simulink model "DIMR_ordinary"  (R2024b)
settings: Solver=daessc  StartTime=0.0  StopTime=60  RelTol=1e-3
values from neighbouring files (symbols this model uses):
  d_m0 = d_mn    (= 0)    [DIMR_main.m]
  d_m_cmd = 0.12787808985686    (= 0.127878089857)    [DIMR_main.m]
  dis_cmd = 0    [DIMR_main.m]
  jrk_cmd = 0.15    [DIMR_main.m]
  phi_cmd = 0*pi/180    (= 0)    [DIMR_main.m]
  ta = (vel_cmd-jrk_cmd*tt^2)/acc_cmd    (= 3.66666666667)    [DIMR_main.m]
  taz = z_vel_cmd/z_acc_cmd    (= 1.6)    [DIMR_main.m]
  tc = (x_cmd-2*(1/2*acc_cmd*ta^2+1/2*jrk_cmd*tt^2*ta+tt*vel_cmd))/vel_cmd    (= 10.6666666667)    [DIMR_main.m]
  tcz = (z_cmd-z_acc_cmd*taz^2)/z_vel_cmd    [DIMR_main.m]
  tcz2 = (z_cmd2-z_acc_cmd*taz^2)/z_vel_cmd    (= 0.9)    [DIMR_main.m]
  theta_f0 = -theta_p0    (= -0.024)    [DIMR_main.m]
  theta_f_cmd = 0.037940459    [DIMR_main.m]
  theta_p0 = theta_pn    (= 0.024)    [DIMR_main.m]
  theta_p_cmd = -0.037940459    [DIMR_main.m]
  ts = 15    [DIMR_main.m]
  ts2 = te+5    (= 39.3333333333)    [DIMR_main.m]
  tsz = 10    [DIMR_main.m]
  tsz2 = ts2    (= 39.3333333333)    [DIMR_main.m]
  tt = acc_cmd/jrk_cmd    (= 0.333333333333)    [DIMR_main.m]
  x_cmd = 3    [DIMR_main.m]
  z_0 = R_wo+L_bmy+L_my/2    [DIMR_main.m]
  z_acc_cmd = 0.05    [DIMR_main.m]
  z_cmd = 0.9-z_0    [DIMR_main.m]
  z_cmd2 = 0.9-0.7    (= 0.2)    [DIMR_main.m]
undefined symbols (not defined in the file or in its folder): Ac, Dc, DiscIntNeverNeededParam, dspblkCoreblockFVToolHelper, g, g_ext, g_fork, g_lift, g_reac, g_spado, g_yaw, gcbh, K_fd, K_fp, K_md, K_mp, K_pd, K_pp, K_wd, K_wi, K_wp, K_yd, K_yp, Kc, L_bg, L_bmx, L_bmy, L_bmz, L_bsx, L_bsy, L_bsz, L_by, L_ex, L_ey, L_ez, L_fg, L_fh, L_fx, L_fy, L_fz, L_lx, L_ly, L_lz, L_mg, L_mx, L_my, L_mz, L_wt, M_b, M_f, M_m, M_n11, M_n21, M_n22, M_n33, M_n44, Mc, N_f, N_w, omega_c ... (+10)
libraries: simulink x56, sm_lib x54, nesl_utility x12, slctrl_autotuning x1, slpidlib x1
(part 6 of 6)

== matlab function DIMR_ordinary/simp_model ==
  data: inv_cog_theta1 output; lt input; mass_l input; tau input; tau_w input; inv_cog_delta2 output; inv_cog_dtheta1 output; inv_cog_ddelta2 output
function [inv_cog_theta1,inv_cog_delta2,inv_cog_dtheta1,inv_cog_ddelta2] = simp_model(lt,mass_l,tau,tau_w)
%#codegen

%    This function was generated by the Symbolic Math Toolbox version 24.2.
%    16-Apr-2025 15:03:53

% lt = complex(lt);  % if required to enforce complex operations
% mass_l = complex(mass_l);  % if required to enforce complex operations
% tau = complex(tau);  % if required to enforce complex operations
% tau_w = complex(tau_w);  % if required to enforce complex operations
t0 = roots([tau.*-4.786091217110344e+34-tau.*tan(atan(((lt.*3.671450002392298e+16-sqrt(lt.^2.*1.34795451200664e+33-tau_w.^2.*3.022314549036573e+27+lt.^2.*tau_w.^2.*4.75626088156714e+29)).*4.447070890666667e+5)./(tau_w.*2.444803076916086e+19-lt.*tau_w.*3.066951346239308e+20)).*2.0).^2.*4.786091217110344e+34-tan(atan(((lt.*3.671450002392298e+16-sqrt(lt.^2.*1.34795451200664e+33-tau_w.^2.*3.022314549036573e+27+lt.^2.*tau_w.^2.*4.75626088156714e+29)).*4.447070890666667e+5)./(tau_w.*2.444803076916086e+19-lt.*tau_w.*3.066951346239308e+20)).*2.0).^2.*1.807017575219593e+35+lt.^2.*tan(atan(((lt.*3.671450002392298e+16-sqrt(lt.^2.*1.34795451200664e+33-tau_w.^2.*3.022314549036573e+27+lt.^2.*tau_w.^2.*4.75626088156714e+29)).*4.447070890666667e+5)./(tau_w.*2.444803076916086e+19-lt.*tau_w.*3.066951346239308e+20)).*2.0).^2.*1.413432750381875e+39-tau.^2.*tan(atan(((lt.*3.671450002392298e+16-sqrt(lt.^2.*1.34795451200664e+33-tau_w.^2.*3.022314549036573e+27+lt.^2.*tau_w.^2.*4.75626088156714e+29)).*4.447070890666667e+5)./(tau_w.*2.444803076916086e+19-lt.*tau_w.*3.066951346239308e+20)).*2.0).^2.*3.169126500570574e+33-tau.^2.*3.169126500570574e+33+lt.^2.*mass_l.*tan(atan(((lt.*3.671450002392298e+16-sqrt(lt.^2.*1.34795451200664e+33-tau_w.^2.*3.022314549036573e+27+lt.^2.*tau_w.^2.*4.75626088156714e+29)).*4.447070890666667e+5)./(tau_w.*2.444803076916086e+19-lt.*tau_w.*3.066951346239308e+20)).*2.0).^2.*4.151050661914464e+37+lt.^2.*mass_l.^2.*tan(atan(((lt.*3.671450002392298e+16-sqrt(lt.^2.*1.34795451200664e+33-tau_w.^2.*3.022314549036573e+27+lt.^2.*tau_w.^2.*4.75626088156714e+29)).*4.447070890666667e+5)./(tau_w.*2.444803076916086e+19-lt.*tau_w.*3.066951346239308e+20)).*2.0).^2.*3.047761132095789e+35-1.807017575219593e+35,lt.^2.*tan(atan(((lt.*3.671450002392298e+16-sqrt(lt.^2.*1.34795451200664e+33-tau_w.^2.*3.022314549036573e+27+lt.^2.*tau_w.^2.*4.75626088156714e+29)).*4.447070890666667e+5)./(tau_w.*2.444803076916086e+19-lt.*tau_w.*3.066951346239308e+20)).*2.0).*5.653731001527501e+39+lt.^2.*mass_l.^2.*tan(atan(((lt.*3.671450002392298e+16-sqrt(lt.^2.*1.34795451200664e+33-tau_w.^2.*3.022314549036573e+27+lt.^2.*tau_w.^2.*4.75626088156714e+29)).*4.447070890666667e+5)./(tau_w.*2.444803076916086e+19-lt.*tau_w.*3.066951346239308e+20)).*2.0).*1.219104452838316e+36+lt.^2.*mass_l.*tan(atan(((lt.*3.671450002392298e+16-sqrt(lt.^2.*1.34795451200664e+33-tau_w.^2.*3.022314549036573e+27+lt.^2.*tau_w.^2.*4.75626088156714e+29)).*4.447070890666667e+5)./(tau_w.*2.444803076916086e+19-lt.*tau_w.*3.066951346239308e+20)).*2.0).*1.660420264765786e+38,tau.*9.572182434220687e+34+tau.*tan(atan(((lt.*3.671450002392298e+16-sqrt(lt.^2.*1.34795451200664e+33-tau_w.^2.*3.022314549036573e+27+lt.^2.*tau_w.^2.*4.75626088156714e+29)).*4.447070890666667e+5)./(tau_w.*2.444803076916086e+19-lt.*tau_w.*3.066951346239308e+20)).*2.0).^2.*9.572182434220687e+34+tan(atan(((lt.*3.671450002392298e+16-sqrt(lt.^2.*1.34795451200664e+33-tau_w.^2.*3.022314549036573e+27+lt.^2.*tau_w.^2.*4.75626088156714e+29)).*4.447070890666667e+5)./(tau_w.*2.444803076916086e+19-lt.*tau_w.*3.066951346239308e+20)).*2.0).^2.*3.614035150439186e+35+lt.^2.*mass_l.*1.660420264765786e+38-lt.^2.*tan(atan(((lt.*3.671450002392298e+16-sqrt(lt.^2.*1.34795451200664e+33-tau_w.^2.*3.022314549036573e+27+lt.^2.*tau_w.^2.*4.75626088156714e+29)).*4.447070890666667e+5)./(tau_w.*2.444803076916086e+19-lt.*tau_w.*3.066951346239308e+20)).*2.0).^2.*2.82686550076375e+39+tau.^2.*tan(atan(((lt.*3.671450002392298e+16-sqrt(lt.^2.*1.34795451200664e+33-tau_w.^2.*3.022314549036573e+27+lt.^2.*tau_w.^2.*4.75626088156714e+29)).*4.447070890666667e+5)./(tau_w.*2.444803076916086e+19-lt.*tau_w.*3.066951346239308e+20)).*2.0).^2.*6.338253001141147e+33+lt.^2.*5.653731001527501e+39+tau.^2.*6.338253001141147e+33+lt.^2.*mass_l.^2.*1.219104452838316e+36-lt.^2.*mass_l.*tan(atan(((lt.*3.671450002392298e+16-sqrt(lt.^2.*1.34795451200664e+33-tau_w.^2.*3.022314549036573e+27+lt.^2.*tau_w.^2.*4.75626088156714e+29)).*4.447070890666667e+5)./(tau_w.*2.444803076916086e+19-lt.*tau_w.*3.066951346239308e+20)).*2.0).^2.*8.302101323828929e+37-lt.^2.*mass_l.^2.*tan(atan(((lt.*3.671450002392298e+16-sqrt(lt.^2.*1.34795451200664e+33-tau_w.^2.*3.022314549036573e+27+lt.^2.*tau_w.^2.*4.75626088156714e+29)).*4.447070890666667e+5)./(tau_w.*2.444803076916086e+19-lt.*tau_w.*3.066951346239308e+20)).*2.0).^2.*6.095522264191578e+35+3.614035150439186e+35,lt.^2.*tan(atan(((lt.*3.671450002392298e+16-sqrt(lt.^2.*1.34795451200664e+33-tau_w.^2.*3.022314549036573e+27+lt.^2.*tau_w.^2.*4.75626088156714e+29)).*4.447070890666667e+5)./(tau_w.*2.444803076916086e+19-lt.*tau_w.*3.066951346239308e+20)).*2.0).*-5.653731001527501e+39-lt.^2.*mass_l.^2.*tan(atan(((lt.*3.671450002392298e+16-sqrt(lt.^2.*1.34795451200664e+33-tau_w.^2.*3.022314549036573e+27+lt.^2.*tau_w.^2.*4.75626088156714e+29)).*4.447070890666667e+5)./(tau_w.*2.444803076916086e+19-lt.*tau_w.*3.066951346239308e+20)).*2.0).*1.219104452838316e+36-lt.^2.*mass_l.*tan(atan(((lt.*3.671450002392298e+16-sqrt(lt.^2.*1.34795451200664e+33-tau_w.^2.*3.022314549036573e+27+lt.^2.*tau_w.^2.*4.75626088156714e+29)).*4.447070890666667e+5)./(tau_w.*2.444803076916086e+19-lt.*tau_w.*3.066951346239308e+20)).*2.0).*1.660420264765786e+38,tau.*-4.786091217110344e+34-tau.*tan(atan(((lt.*3.671450002392298e+16-sqrt(lt.^2.*1.34795451200664e+33-tau_w.^2.*3.022314549036573e+27+lt.^2.*tau_w.^2.*4.75626088156714e+29)).*4.447070890666667e+5)./(tau_w.*2.444803076916086e+19-lt.*tau_w.*3.066951346239308e+20)).*2.0).^2.*4.786091217110344e+34-tan(atan(((lt.*3.671450002392298e+16-sqrt(lt.^2.*1.34795451200664e+33-tau_w.^2.*3.022314549036573e+27+lt.^2.*tau_w.^2.*4.75626088156714e+29)).*4.447070890666667e+5)./(tau_w.*2.444803076916086e+19-lt.*tau_w.*3.066951346239308e+20)).*2.0).^2.*1.807017575219593e+35+lt.^2.*tan(atan(((lt.*3.671450002392298e+16-sqrt(lt.^2.*1.34795451200664e+33-tau_w.^2.*3.022314549036573e+27+lt.^2.*tau_w.^2.*4.75626088156714e+29)).*4.447070890666667e+5)./(tau_w.*2.444803076916086e+19-lt.*tau_w.*3.066951346239308e+20)).*2.0).^2.*1.413432750381875e+39-tau.^2.*tan(atan(((lt.*3.671450002392298e+16-sqrt(lt.^2.*1.34795451200664e+33-tau_w.^2.*3.022314549036573e+27+lt.^2.*tau_w.^2.*4.75626088156714e+29)).*4.447070890666667e+5)./(tau_w.*2.444803076916086e+19-lt.*tau_w.*3.066951346239308e+20)).*2.0).^2.*3.169126500570574e+33-tau.^2.*3.169126500570574e+33+lt.^2.*mass_l.*tan(atan(((lt.*3.671450002392298e+16-sqrt(lt.^2.*1.34795451200664e+33-tau_w.^2.*3.022314549036573e+27+lt.^2.*tau_w.^2.*4.75626088156714e+29)).*4.447070890666667e+5)./(tau_w.*2.444803076916086e+19-lt.*tau_w.*3.066951346239308e+20)).*2.0).^2.*4.151050661914464e+37+lt.^2.*mass_l.^2.*tan(atan(((lt.*3.671450002392298e+16-sqrt(lt.^2.*1.34795451200664e+33-tau_w.^2.*3.022314549036573e+27+lt.^2.*tau_w.^2.*4.75626088156714e+29)).*4.447070890666667e+5)./(tau_w.*2.444803076916086e+19-lt.*tau_w.*3.066951346239308e+20)).*2.0).^2.*3.047761132095789e+35-1.807017575219593e+35]);
if tau_w >= 0
    t2 = real(t0(4));
else
    t2 = real(t0(3));
end
inv_cog_theta1 = atan(t2).*2.0;
if nargout > 1
    t3 = lt.^2;
    t4 = mass_l.^2;
    t5 = t2.^2;
    t6 = t2.^3;
    t7 = tau.^2;
    t8 = tau_w.^2;
    t9 = tau_w.*4.0e+2;
    t10 = lt.*3.671450002392298e+16;
    t14 = lt.*tau_w.*5.017911463213649e+3;
    t11 = t8.*3.022314549036573e+27;
    t13 = t3.*1.34795451200664e+33;
    t15 = -t14;
    t18 = t3.*t8.*4.75626088156714e+29;
    t12 = -t11;
    t16 = t9+t15;
    t17 = 1.0./t16;
    t19 = t12+t13+t18;
    t20 = sqrt(t19);
    t21 = -t20;
    t22 = t10+t21;
    t23 = (t17.*t22)./1.37438953472e+11;
    t24 = atan(t23);
    t25 = t24.*2.0;
    t26 = tan(t25);
    t27 = t26.^2;
    t28 = t26.^3;
    et1 = mass_l.*7.462747908049749e+36+t2.*2.168421090263512e+37-t6.*7.228070300878373e+36+t26.*7.228070300878373e+36;
    et2 = t27.*3.210929424600914e+38+t28.*7.228070300878373e+36+tau.*4.252255575316159e+37+mass_l.*t27.*7.462747908049749e+36;
    et3 = mass_l.*tau.*9.882967578188891e+35+t2.*t3.*2.261492400611e+41+t2.*t7.*3.802951800684688e+35-t6.*t7.*1.267650600228229e+35;
    et4 = t2.*t27.*2.168421090263512e+37-t3.*t26.*1.1307462003055e+41-t3.*t28.*5.653731001527501e+40-t5.*t26.*7.228070300878373e+36;
    et5 = t5.*t28.*-7.228070300878373e+36-t6.*t27.*7.228070300878373e+36+t7.*t26.*1.267650600228229e+35+t7.*t28.*1.267650600228229e+35;
    et6 = tau.*t2.*5.743309460532412e+36-t6.*tau.*1.914436486844137e+36+t26.*tau.*1.914436486844137e+36+t27.*tau.*4.252255575316159e+37;
    et7 = t28.*tau.*1.914436486844137e+36+mass_l.*t2.*t3.*6.641681059063143e+39-mass_l.*t3.*t26.*3.320840529531572e+39-mass_l.*t3.*t28.*1.660420264765786e+39;
    et8 = mass_l.*t27.*tau.*9.882967578188891e+35+t2.*t3.*t4.*4.876417811353262e+37+t2.*t3.*t27.*5.653731001527501e+40-t3.*t4.*t26.*2.438208905676631e+37;
    et9 = t3.*t5.*t26.*2.261492400611e+41-t3.*t4.*t28.*1.219104452838316e+37+t2.*t7.*t27.*3.802951800684688e+35+t3.*t5.*t28.*5.653731001527501e+40;
    et10 = t3.*t6.*t27.*5.653731001527501e+40-t5.*t7.*t26.*1.267650600228229e+35-t5.*t7.*t28.*1.267650600228229e+35-t6.*t7.*t27.*1.267650600228229e+35;
    et11 = t2.*t27.*tau.*5.743309460532412e+36-t5.*t26.*tau.*1.914436486844137e+36-t5.*t28.*tau.*1.914436486844137e+36-t6.*t27.*tau.*1.914436486844137e+36;
    et12 = mass_l.*t2.*t3.*t27.*1.660420264765786e+39+mass_l.*t3.*t5.*t26.*6.641681059063143e+39+mass_l.*t3.*t5.*t28.*1.660420264765786e+39+mass_l.*t3.*t6.*t27.*1.660420264765786e+39;
    et13 = t2.*t3.*t4.*t27.*1.219104452838316e+37+t3.*t4.*t5.*t26.*4.876417811353262e+37+t3.*t4.*t5.*t28.*1.219104452838316e+37+t3.*t4.*t6.*t27.*1.219104452838316e+37;
    et14 = 3.210929424600914e+38;
    inv_cog_delta2 = ((et1+et2+et3+et4+et5+et6+et7+et8+et9+et10+et11+et12+et13+et14).*(-2.264224836463332e-20))./((mass_l+2.5e+1).*(tau.*5.62949953421312e+16+4.250902933753714e+17).*(t27+1.0));
end
if nargout > 2
    inv_cog_dtheta1 = 0.0;
end
if nargout > 3
    inv_cog_ddelta2 = 0.0;
end
end

== stateflow chart DIMR_ordinary/Chart ==
  state Change_Height_1
    entry:
    [theta1,delta2,dtheta1,ddelta2,lt] = IK(dz,tau,z)
    during:
    [theta1,delta2,dtheta1,ddelta2,lt] = IK(dz,tau,z)
  state Move
    entry:
    [theta1,delta2,dtheta1,ddelta2] = simp_model(lt,tau,tau_w)
    during:
    [theta1,delta2,dtheta1,ddelta2] = simp_model(lt,tau,tau_w)
  (default) -> Change_Height_1
  Change_Height_1 -> Move : [abs(z_curr - z_cmd)<=0.001]
  data: dz function_input; tau function_input; z function_input; ik_theta1 function_output; ik_delta2 function_output; ik_dtheta1 function_output; ik_ddelta2 function_output; ik_lt function_output; lt function_input; tau function_input; tau_w function_input; inv_cog_theta1 function_output; inv_cog_delta2 function_output; inv_cog_dtheta1 function_output; inv_cog_ddelta2 function_output; tau_w input; z input; dz input; z_curr input; ddelta2 output; delta2 output; dtheta1 output; theta1 output; lt local; z_cmd input double; tau input
  function [ik_theta1,ik_delta2,ik_dtheta1,ik_ddelta2,ik_lt] = IK(dz,tau,z):
    | function [ik_theta1,ik_delta2,ik_dtheta1,ik_ddelta2,ik_lt] = IK(dz,tau,z)
    | %#codegen
    | 
    | %    This function was generated by the Symbolic Math Toolbox version 24.2.
    | %    15-Apr-2025 18:25:07
    | 
    | % dz = complex(dz);  % if required to enforce complex operations
    | % tau = complex(tau);  % if required to enforce complex operations
    | % z = complex(z);  % if required to enforce complex operations
    | t0 = roots([1.0,(tau.*8.44424930131968e+16-z.*6.07271847679102e+19-tau.*z.*1.125899906842624e+18+2.195986091984785e+19)./(tau.*1.238489897526886e+17+9.351986454258171e+17),0.0,((tau.*-8.44424930131968e+16+z.*6.07271847679102e+19+tau.*z.*1.125899906842624e+18+1.285078320466132e+19).*(-1.0./4.4e+2))./(tau.*2.81474976710656e+14+2.125451466876857e+15),-1.0]);
    | t2 = real(t0(4));
    | t3 = atan2(t2,1);
    | t4 = t2.^2;
    | t5 = t2.^3;
    | t6 = tau.^2;
    | t7 = tau.^3;
    | t9 = tau.^5;
    | t11 = z.^2;
    | t12 = z.^3;
    | t14 = z.^5;
    | t19 = tau.*1.40737488355328e+14;
    | t20 = tau.*5.319877059831398e+17;
    | t21 = t2.*tau.*1.238489897526886e+17;
    | t22 = t2.*9.351986454258171e+17;
    | t23 = tau.*z.*1.125899906842624e+18;
    | t24 = z.*6.07271847679102e+19;
    | t35 = tau.*4.635073695354219e-1;
    | t57 = tau.*5.743900035854321e+113;
    | t66 = tau.*z.*7.990597029423474e+114;
    | t74 = z.*1.447317376015955e+116;
    | t8 = t6.^2;
    | t10 = t6.^3;
    | t13 = t11.^2;
    | t15 = t11.^3;
    | t16 = t3.*2.0;
    | ik_theta1 = t16;
    | if nargout > 1
    |     t25 = -t23;
    |     t26 = -t24;
    |     t27 = t4.*tau.*8.44424930131968e+16;
    |     t28 = t5.*tau.*1.238489897526886e+17;
    |     t29 = t5.*9.351986454258171e+17;
    |     t30 = t4.*2.195986091984785e+19;
    |     t33 = t4.*tau.*z.*-1.125899906842624e+18;
    |     t34 = t4.*z.*-6.07271847679102e+19;
    |     t36 = t19+7.590898095988775e+15;
    |     t38 = t35+7.0./2.0;
    |     t39 = t35+6.81e+2./1.0e+1;
    |     t42 = t9.*2.386050182016105e+106;
    |     t46 = t9.*z.*4.211088297564564e+107;
    |     t51 = t7.*2.507343178421252e+110;
    |     t52 = t9.*t11.*4.593987726794744e+108;
    |     t58 = t9.*t12.*2.604615627247899e+109;
    |     t60 = t6.*2.999842761429269e+112;
    |     t61 = t7.*z.*9.409126505705104e+111;
    |     t65 = t9.*t14.*2.966510080312107e+110;
    |     t72 = -t66;
    |     t73 = t6.*z.*3.660741181676567e+113;
    |     t75 = t7.*t11.*6.407841099867219e+112;
    |     t76 = t7.*t12.*3.958710038416369e+112;
    |     t81 = -t74;
    |     t86 = t11.*tau.*3.585353509436109e+115;
    |     t87 = t6.*t11.*2.09113906624741e+114;
    |     t88 = t6.*t12.*3.785302651403782e+114;
    |     t90 = t7.*t14.*2.876678343420641e+114;
    |     t92 = t11.*7.09032593341523e+116;
    |     t93 = t12.*tau.*2.133985804221304e+116;
    |     t95 = t12.*3.242008287042286e+117;
    |     t98 = t14.*2.256895254686051e+118;
    |     t101 = t14.*tau.*2.510610198759619e+117;
    |     t102 = t6.*t14.*1.163686329155874e+116;
    |     t17 = cos(t16);
    |     t18 = sin(t16);
    |     t37 = 1.0./t36;
    |     t40 = 1.0./t39.^2;
    |     t41 = t10.*3.212055390272792e+104;
    |     t43 = t10.*z.*2.675474179773727e+105;
    |     t44 = t8.*2.477746168797788e+107;
    |     t47 = t10.*t11.*2.526492816377412e+106;
    |     t48 = -t46;
    |     t49 = t10.*t12.*1.059207781794524e+107;
    |     t50 = t10.*t13.*4.676525342669896e+107;
    |     t54 = t10.*t14.*9.166661893505187e+107;
    |     t55 = t10.*t15.*2.037035976334486e+108;
    |     t56 = t8.*z.*9.736596647488009e+109;
    |     t63 = -t58;
    |     t64 = t9.*t13.*1.239018969121646e+110;
    |     t67 = -t61;
    |     t68 = t8.*t11.*7.882227863274746e+110;
    |     t69 = t8.*t12.*2.154890938178742e+111;
    |     t70 = -t65;
    |     t71 = t9.*t15.*6.592244622915794e+110;
    |     t78 = t8.*t13.*1.21830758387732e+112;
    |     t79 = t8.*t14.*4.00008483587525e+112;
    |     t80 = -t73;
    |     t82 = -t76;
    |     t83 = t7.*t13.*4.915417942081258e+113;
    |     t85 = t8.*t15.*8.88907741305611e+112;
    |     t89 = t6.*t13.*1.928403609769147e+114;
    |     t91 = t7.*t15.*6.392618540934758e+114;
    |     t94 = t13.*tau.*3.97502326562149e+116;
    |     t96 = -t90;
    |     t97 = t13.*7.985575221783389e+117;
    |     t99 = t15.*5.015322788191225e+118;
    |     t103 = t6.*t15.*2.585969620346386e+116;
    |     t105 = -t98;
    |     t106 = -t101;
    |     t107 = t15.*tau.*5.579133775021375e+117;
    |     t108 = -t102;
    |     t109 = t20+t21+t22+t25+t26+t27+t28+t29+t30+t33+t34+2.869359480283757e+19;
    |     t45 = -t43;
    |     t53 = -t49;
    |     t59 = -t54;
    |     t62 = -t56;
    |     t77 = -t69;
    |     t84 = -t79;
    |     t100 = -t94;
    |     t104 = -t97;
    |     t110 = (t37.*t109)./8.0e+3;
    |     ik_delta2 = -t110;
    | end
    | if nargout > 2
    |     t111 = t110-1.59e+2./4.0e+2;
    |     t112 = t41+t42+t44+t45+t47+t48+t50+t51+t52+t53+t55+t57+t59+t60+t62+t63+t64+t67+t68+t70+t71+t72+t75+t77+t78+t80+t81+t82+t83+t84+t85+t86+t87+t88+t89+t91+t92+t93+t95+t96+t99+t100+t103+t104+t105+t106+t107+t108-2.105477541297374e+115;
    |     t113 = 1.0./t112;
    |     et1 = t2.*-1.753894605876528e+96+t4.*1.009464978528226e+96;
    |     et2 = t5.*4.619988807297373e+94-t6.*2.554852704393891e+92;
    |     et3 = t7.*-7.8111064788263e+89-t8.*1.00794759003273e+89;
    |     et4 = t9.*1.814387972119789e+86+t11.*6.245124509053326e+96;
    |     et5 = t12.*-3.331857083120826e+97;
    |     et6 = t13.*3.815554989087441e+97-tau.*5.24829876676123e+94;
    |     et7 = z.*1.399328629129073e+96-t2.*t6.*1.075720720231548e+91;
    |     et8 = t2.*t7.*-1.388092428471541e+90+t2.*t8.*7.128076116355089e+88;
    |     et9 = t4.*t6.*1.722969069981006e+93+t2.*t9.*1.361707336651519e+86;
    |     et10 = t4.*t7.*-1.973567476521639e+90+t5.*t6.*9.078257330103773e+92;
    |     et11 = t4.*t8.*1.151036106739522e+89+t5.*t7.*6.111449310419045e+90;
    |     et12 = t2.*t11.*5.875732481208788e+97+t4.*t9.*1.343184695804828e+87;
    |     et13 = t5.*t8.*-2.551325158332646e+88-t2.*t12.*1.782863198738202e+97;
    |     et14 = t5.*t9.*5.322204718218049e+86-t2.*t13.*5.464130766461227e+98;
    |     et15 = t4.*t11.*4.415911382468272e+97;
    |     et16 = t2.*t14.*8.258777032656798e+98;
    |     et17 = t4.*t12.*-8.469349253727501e+97;
    |     et18 = t5.*t11.*9.380726613532944e+95;
    |     et19 = t4.*t13.*6.359258315145734e+97;
    |     et20 = t5.*t12.*-1.175190936638932e+96+t6.*t11.*5.907708747848193e+94;
    |     et21 = t6.*t12.*-3.196898258866477e+95+t7.*t11.*1.247609721739556e+93;
    |     et22 = t6.*t13.*4.534279766579717e+95-t7.*t12.*6.544610701214467e+93;
    |     et23 = t8.*t11.*1.242487226117768e+91+t7.*t13.*1.139418916775499e+94;
    |     et24 = t8.*t12.*-5.845583673798496e+91+t9.*t11.*4.904790067467224e+88;
    |     et25 = t8.*t13.*1.333203858988986e+92-t9.*t12.*1.791158880389735e+89;
    |     et26 = t9.*t13.*5.970529601299116e+89+tau.*t2.*1.323988270291723e+93;
    |     et27 = t4.*tau.*1.468522013529346e+95+t5.*tau.*1.261219729665987e+94;
    |     et28 = t11.*tau.*1.207196483550789e+96;
    |     et29 = t12.*tau.*-6.477833809662083e+96;
    |     et30 = t13.*tau.*7.882625873837409e+96;
    |     et31 = z.*t2.*-1.890970205684437e+96;
    |     et32 = t4.*z.*-1.069218722198518e+97;
    |     et33 = t5.*z.*-3.150739272925472e+95+t6.*z.*2.668557352126731e+93;
    |     et34 = t7.*z.*4.092978643690637e+91+t8.*z.*6.846342443053817e+89;
    |     et35 = t9.*z.*-5.342131360762384e+87+tau.*z.*2.034429880145039e+95;
    |     et36 = t2.*t6.*t11.*3.834597488658114e+94+t2.*t6.*t12.*1.79267290146031e+95;
    |     et37 = t2.*t7.*t11.*3.241447763154754e+92-t2.*t6.*t13.*1.552786419763549e+96;
    |     et38 = t2.*t7.*t12.*4.397794916127146e+93+t2.*t8.*t11.*6.696326945473049e+89;
    |     et39 = t4.*t6.*t11.*2.979273638991897e+95;
    |     et40 = t2.*t6.*t14.*2.838892916716577e+96;
    |     et41 = t2.*t7.*t13.*-2.577198424443163e+94+t2.*t8.*t12.*4.358240682659937e+91;
    |     et42 = t2.*t9.*t11.*-1.748415316198616e+88-t4.*t6.*t12.*7.776982869967544e+95;
    |     et43 = t4.*t7.*t11.*4.360273950273173e+93+t5.*t6.*t11.*2.746751487155486e+94;
    |     et44 = t2.*t7.*t14.*5.263391152880169e+94-t2.*t8.*t13.*2.109408183024797e+92;
    |     et45 = t2.*t9.*t12.*1.455542746740951e+89+t4.*t6.*t13.*7.557132944299528e+95;
    |     et46 = t4.*t7.*t12.*-1.507615643654141e+94+t4.*t8.*t11.*2.876061807193666e+91;
    |     et47 = t5.*t6.*t12.*-3.913495645809803e+94+t5.*t7.*t11.*8.312588465463616e+92;
    |     et48 = t2.*t8.*t14.*4.879241176214998e+92-t2.*t9.*t13.*6.784692728748996e+89;
    |     et49 = t4.*t7.*t13.*1.899031527959165e+94-t4.*t8.*t12.*1.220393558543954e+92;
    |     et50 = t4.*t9.*t11.*1.010114099713122e+89-t5.*t7.*t12.*1.474838834239447e+93;
    |     et51 = t5.*t8.*t11.*9.289616355673145e+90+t2.*t9.*t14.*1.809251394333066e+90;
    |     et52 = t4.*t8.*t13.*2.22200643164831e+92-t4.*t9.*t12.*2.985264800649558e+89;
    |     et53 = t5.*t8.*t12.*-2.32376788561945e+91+t5.*t9.*t11.*2.955412152643063e+88;
    |     et54 = t4.*t9.*t13.*9.950882668831861e+89-t5.*t9.*t12.*1.313516512285806e+89;
    |     et55 = t2.*t11.*tau.*2.467684994491885e+96;
    |     et56 = t2.*t12.*tau.*2.151307797149133e+96;
    |     et57 = t2.*t13.*tau.*-4.626464408073966e+97;
    |     et58 = t4.*t11.*tau.*7.861141246672502e+96;
    |     et59 = t2.*t14.*tau.*7.65600803597262e+97;
    |     et60 = t4.*t12.*tau.*-1.628045107945128e+97;
    |     et61 = t5.*t11.*tau.*2.881458695288517e+95;
    |     et62 = t4.*t13.*tau.*1.313770978972902e+97;
    |     et63 = t5.*t12.*tau.*-3.766278218797084e+95-t2.*t6.*z.*8.69453683410162e+92;
    |     et64 = t2.*t7.*z.*-8.14011166039339e+90-t2.*t8.*z.*7.354331859382801e+89;
    |     et65 = t4.*t6.*z.*-4.607531607862968e+94-t2.*t9.*z.*1.094057710499569e+87;
    |     et66 = t4.*t7.*z.*-4.316771097086506e+92-t5.*t6.*z.*7.922329257005371e+93;
    |     et67 = t4.*t8.*z.*-2.629642166088229e+90-t5.*t7.*z.*1.751142096260925e+92;
    |     et68 = t4.*t9.*z.*-1.179328859496608e+88-t5.*t8.*z.*1.536226654469186e+90;
    |     et69 = t5.*t9.*z.*-8.573979033945596e+87-tau.*z.*t2.*1.644111357410597e+95;
    |     et70 = t4.*tau.*z.*-1.740373755123545e+96;
    |     et71 = t5.*tau.*z.*-9.219656825165702e+94-3.817418975922806e+95;
    |     ik_dtheta1 = dz.*t36.*t113.*(et1+et2+et3+et4+et5+et6+et7+et8+et9+et10+et11+et12+et13+et14+et15+et16+et17+et18+et19+et20+et21+et22+et23+et24+et25+et26+et27+et28+et29+et30+et31+et32+et33+et34+et35+et36+et37+et38+et39+et40+et41+et42+et43+et44+et45+et46+et47+et48+et49+et50+et51+et52+et53+et54+et55+et56+et57+et58+et59+et60+et61+et62+et63+et64+et65+et66+et67+et68+et69+et70+et71).*8.0e+3;
    | end
    | if nargout > 3
    |     et72 = t2.*-3.7071702195569e+114;
    |     et73 = t4.*3.804188113277026e+115;
    |     et74 = t5.*1.625202646823668e+114;
    |     et75 = t6.*1.140152959101139e+112;
    |     et76 = t7.*3.851536071140141e+109;
    |     et77 = t8.*4.771323709725432e+107;
    |     et78 = t9.*2.37036597763644e+105;
    |     et79 = t10.*3.344342724717159e+103;
    |     et80 = t11.*6.661710042517029e+116;
    |     et81 = t12.*3.317645224682185e+117;
    |     et82 = t13.*-8.033152579881287e+117+t55+t59+t70+t71+t84+t85+t91+t96+t99+t103+t105+t106+t107+t108;
    |     et83 = tau.*3.305389407105682e+113;
    |     et84 = z.*-1.344576683503948e+116;
    |     et85 = t2.*t6.*-5.521484071666565e+111;
    |     et86 = t2.*t7.*-1.201004210046715e+109;
    |     et87 = t2.*t8.*-1.446897405085628e+108;
    |     et88 = t4.*t6.*-7.600317735708989e+111;
    |     et89 = t2.*t9.*-6.836757611015585e+105;
    |     et90 = t4.*t7.*9.237917051294251e+109;
    |     et91 = t5.*t6.*-8.407795288014511e+110;
    |     et92 = t2.*t10.*4.905035996251834e+103;
    |     et93 = t4.*t8.*6.21766718480593e+107;
    |     et94 = t5.*t7.*-1.679675237605966e+109;
    |     et95 = t2.*t11.*2.425689270038724e+115;
    |     et96 = t4.*t9.*-2.369824972154481e+105;
    |     et97 = t5.*t8.*1.018828318361818e+108;
    |     et98 = t2.*t12.*-6.307571438901966e+116;
    |     et99 = t4.*t10.*3.344342724717159e+103;
    |     et100 = t5.*t9.*7.067802508371117e+105;
    |     et101 = t2.*t13.*1.396484281539863e+117;
    |     et102 = t4.*t11.*-1.402659673535802e+117;
    |     et103 = t5.*t10.*4.905035996251834e+103;
    |     et104 = t2.*t14.*-7.723597093814486e+116;
    |     et105 = t4.*t12.*3.938271388021781e+117;
    |     et106 = t5.*t11.*-5.533248821789028e+115;
    |     et107 = t4.*t13.*1.098783857622504e+118;
    |     et108 = t5.*t12.*1.557427551233363e+115;
    |     et109 = t6.*t11.*7.991271506884402e+113;
    |     et110 = t4.*t14.*-5.131828736560907e+118;
    |     et111 = t5.*t13.*5.110047691224071e+116;
    |     et112 = t6.*t12.*6.388892406797049e+114;
    |     et113 = t7.*t11.*2.225465716458933e+112;
    |     et114 = t5.*t14.*-7.723597093814486e+116;
    |     et115 = t6.*t13.*6.133630224665161e+112;
    |     et116 = t7.*t12.*6.414800515945154e+112;
    |     et117 = t8.*t11.*2.190420013370623e+110;
    |     et118 = t7.*t13.*4.024585580613185e+113;
    |     et119 = t8.*t12.*-3.271771400537028e+110;
    |     et120 = t9.*t11.*9.648630921792687e+107;
    |     et121 = t8.*t13.*1.013528935640283e+112;
    |     et122 = t9.*t12.*-1.235951960272058e+109;
    |     et123 = t10.*t11.*1.239367190298751e+106;
    |     et124 = t9.*t13.*1.011419526100604e+110;
    |     et125 = t10.*t12.*-7.63430158030757e+106;
    |     et126 = t10.*t13.*3.690599930124005e+107+t4.*t55+t4.*t71+t4.*t85+t4.*t91+t4.*t99+t4.*t103+t4.*t107;
    |     et127 = tau.*t2.*-5.325511928164662e+113;
    |     et128 = t4.*tau.*-4.601389533003556e+111;
    |     et129 = t5.*tau.*2.102524928619955e+113;
    |     et130 = t11.*tau.*2.257239068666816e+115;
    |     et131 = t12.*tau.*2.379035049732175e+116;
    |     et132 = t13.*tau.*-4.136321230248881e+116;
    |     et133 = z.*t2.*3.113201852556033e+115;
    |     et134 = t4.*z.*-6.511422436340579e+115;
    |     et135 = t5.*z.*1.662776353932113e+114;
    |     et136 = t6.*z.*-9.989623857325219e+112;
    |     et137 = t7.*z.*-3.096673052545432e+111;
    |     et138 = t8.*z.*-3.937587938067827e+109;
    |     et139 = t9.*z.*-6.92947223565074e+106;
    |     et140 = t10.*z.*-1.077535567389974e+105;
    |     et141 = tau.*z.*-4.956122630630957e+114;
    |     et142 = t2.*t6.*t11.*5.463288101128978e+113;
    |     et143 = t2.*t6.*t12.*-6.870842133918736e+114;
    |     et144 = t2.*t7.*t11.*1.493465513298907e+112;
    |     et145 = t2.*t6.*t13.*1.770473980809039e+115;
    |     et146 = t2.*t7.*t12.*-1.662839869670821e+113;
    |     et147 = t2.*t8.*t11.*1.600464698420783e+110;
    |     et148 = t4.*t6.*t11.*-1.185362385403583e+114;
    |     et149 = t2.*t6.*t14.*-1.213681741815904e+115;
    |     et150 = t2.*t7.*t13.*4.808389969487753e+113;
    |     et151 = t2.*t8.*t12.*-2.039300901034873e+111;
    |     et152 = t2.*t9.*t11.*9.085779705955538e+107;
    |     et153 = t4.*t6.*t12.*1.484825663584366e+113;
    |     et154 = t4.*t7.*t11.*-6.414166966086719e+111;
    |     et155 = t5.*t6.*t11.*-3.653957848263659e+113;
    |     et156 = t2.*t7.*t14.*-4.008171825166093e+113;
    |     et157 = t2.*t8.*t13.*6.483084785515751e+111;
    |     et158 = t2.*t9.*t12.*-1.26913217775301e+109;
    |     et159 = t2.*t10.*t11.*5.825642799869884e+105;
    |     et160 = t4.*t6.*t13.*5.411483176200627e+115;
    |     et161 = t4.*t7.*t12.*-8.894206859842618e+112;
    |     et162 = t4.*t8.*t11.*5.436080491457138e+109;
    |     et163 = t5.*t6.*t12.*-5.173317577586963e+113;
    |     et164 = t5.*t7.*t11.*-6.429724676055676e+111;
    |     et165 = t2.*t8.*t14.*-6.974962743444695e+111;
    |     et166 = t2.*t9.*t13.*4.061517620170128e+109;
    |     et167 = t2.*t10.*t12.*-3.429451917957924e+106;
    |     et168 = t4.*t6.*t14.*-2.15192323946998e+116;
    |     et169 = t4.*t7.*t13.*1.299597929976685e+114;
    |     et170 = t4.*t8.*t12.*-1.844308794184032e+111;
    |     et171 = t4.*t9.*t11.*1.573497725719581e+108;
    |     et172 = t5.*t6.*t13.*7.181993187065789e+114;
    |     et173 = t5.*t7.*t12.*-3.254097673006372e+112;
    |     et174 = t5.*t8.*t11.*-6.043433221327569e+109;
    |     et175 = t2.*t9.*t14.*-6.212091849660983e+109;
    |     et176 = t2.*t10.*t13.*8.402773402379755e+106;
    |     et177 = t4.*t7.*t14.*-4.708898706530657e+114;
    |     et178 = t4.*t8.*t13.*1.74782751136632e+112;
    |     et179 = t4.*t9.*t12.*-1.742635765920156e+109;
    |     et180 = t4.*t10.*t11.*1.239367190298751e+106;
    |     et181 = t5.*t6.*t14.*-1.213681741815904e+115;
    |     et182 = t5.*t7.*t13.*2.164129541447379e+113;
    |     et183 = t5.*t8.*t12.*-7.898098107882316e+110;
    |     et184 = t5.*t9.*t11.*1.056305699482443e+107;
    |     et185 = t2.*t10.*t14.*-2.240739573967935e+107;
    |     et186 = t4.*t8.*t14.*-5.698580117703968e+112;
    |     et187 = t4.*t9.*t13.*1.247599050175231e+110;
    |     et188 = t4.*t10.*t12.*-7.63430158030757e+106;
    |     et189 = t5.*t7.*t14.*-4.008171825166093e+113;
    |     et190 = t5.*t8.*t13.*3.389105780136559e+111;
    |     et191 = t5.*t9.*t12.*-8.534562153816679e+108;
    |     et192 = t5.*t10.*t11.*5.825642799869884e+105;
    |     et193 = t4.*t9.*t14.*-3.596322144511111e+110;
    |     et194 = t4.*t10.*t13.*3.690599930124005e+107;
    |     et195 = t5.*t8.*t14.*-6.974962743444695e+111;
    |     et196 = t5.*t9.*t13.*2.67593107893232e+109;
    |     et197 = t5.*t10.*t12.*-3.429451917957924e+106;
    |     et198 = t4.*t10.*t14.*-9.166661893505187e+107;
    |     et199 = t5.*t9.*t14.*-6.212091849660983e+109;
    |     et200 = t5.*t10.*t13.*8.402773402379755e+106;
    |     et201 = t5.*t10.*t14.*-2.240739573967935e+107;
    |     et202 = t2.*t11.*tau.*6.55228474510829e+114;
    |     et203 = t2.*t12.*tau.*-1.267703580425692e+116;
    |     et204 = t2.*t13.*tau.*2.938721960462308e+116;
    |     et205 = t4.*t11.*tau.*-7.04099589462565e+115;
    |     et206 = t2.*t14.*tau.*-1.738830026548328e+116;
    |     et207 = t4.*t12.*tau.*1.630150948443772e+116;
    |     et208 = t5.*t11.*tau.*-9.746468343421371e+114;
    |     et209 = t4.*t13.*tau.*1.19686993761682e+117;
    |     et210 = t5.*t12.*tau.*-3.016101165989628e+113;
    |     et211 = t4.*t14.*tau.*-5.175715910305871e+117;
    |     et212 = t5.*t13.*tau.*1.10939340005696e+116;
    |     et213 = t5.*t14.*tau.*-1.738830026548328e+116;
    |     et214 = t2.*t6.*z.*8.794648178204421e+112;
    |     et215 = t2.*t7.*z.*7.919641221873595e+110;
    |     et216 = t2.*t8.*z.*1.21602593543738e+109;
    |     et217 = t4.*t6.*z.*2.781622178886485e+112;
    |     et218 = t2.*t9.*z.*-2.896086435720579e+106;
    |     et219 = t4.*t7.*z.*-2.055401707707991e+110;
    |     et220 = t5.*t6.*z.*1.514114329663636e+112;
    |     et221 = t2.*t10.*z.*-9.263806993383842e+104;
    |     et222 = t4.*t8.*z.*7.430651182143457e+108;
    |     et223 = t5.*t7.*z.*-1.961418471770079e+110;
    |     et224 = t4.*t9.*z.*-3.120986874463163e+106;
    |     et225 = t5.*t8.*z.*-1.733280133320865e+108;
    |     et226 = t4.*t10.*z.*-1.077535567389974e+105;
    |     et227 = t5.*t9.*z.*4.471769997311462e+106;
    |     et228 = t5.*t10.*z.*-9.263806993383842e+104;
    |     et229 = tau.*z.*t2.*4.747078578574793e+114;
    |     et230 = t4.*tau.*z.*1.829231727498887e+114;
    |     et231 = t5.*tau.*z.*3.448046785767965e+113;
    |     et232 = -2.19283328574275e+115;
    |     ik_ddelta2 = dz.*t113.*(et72+et73+et74+et75+et76+et77+et78+et79+et80+et81+et82+et83+et84+et85+et86+et87+et88+et89+et90+et91+et92+et93+et94+et95+et96+et97+et98+et99+et100+et101+et102+et103+et104+et105+et106+et107+et108+et109+et110+et111+et112+et113+et114+et115+et116+et117+et118+et119+et120+et121+et122+et123+et124+et125+et126+et127+et128+et129+et130+et131+et132+et133+et134+et135+et136+et137+et138+et139+et140+et141+et142+et143+et144+et145+et146+et147+et148+et149+et150+et151+et152+et153+et154+et155+et156+et157+et158+et159+et160+et161+et162+et163+et164+et165+et166+et167+et168+et169+et170+et171+et172+et173+et174+et175+et176+et177+et178+et179+et180+et181+et182+et183+et184+et185+et186+et187+et188+et189+et190+et191+et192+et193+et194+et195+et196+et197+et198+et199+et200+et201+et202+et203+et204+et205+et206+et207+et208+et209+et210+et211+et212+et213+et214+et215+et216+et217+et218+et219+et220+et221+et222+et223+et224+et225+et226+et227+et228+et229+et230+et231+et232);
    | end
    | if nargout > 4
    |     ik_lt = sqrt(t40.*(t17.*7.165375-t17.*t111.*(4.3e+1./2.0)+t38.*(t17.*(1.59e+2./4.0e+2)-(t17.*t37.*t109)./8.0e+3)).^2+t40.*(t18.*7.165375-t18.*t111.*(4.3e+1./2.0)+t38.*(t18.*(1.59e+2./4.0e+2)-(t18.*t37.*t109)./8.0e+3+1.1e+1./5.0e+1)).^2);
    | end
    | end
  function [inv_cog_theta1,inv_cog_delta2,inv_cog_dtheta1,inv_cog_ddelta2] = simp_model(lt,tau,tau_w):
    | function [inv_cog_theta1,inv_cog_delta2,inv_cog_dtheta1,inv_cog_ddelta2] = simp_model(lt,tau,tau_w)
    | %#codegen
    | 
    | %    This function was generated by the Symbolic Math Toolbox version 24.2.
    | %    15-Apr-2025 18:25:12
    | 
    | % lt = complex(lt);  % if required to enforce complex operations
    | % tau = complex(tau);  % if required to enforce complex operations
    | % tau_w = complex(tau_w);  % if required to enforce complex operations
    | t0 = roots([tau.*-1.447792593175879e+32-tau.*tan(atan(((lt.*3.671450002392298e+16-sqrt(lt.^2.*1.34795451200664e+33-tau_w.^2.*3.022314549036573e+27+lt.^2.*tau_w.^2.*4.75626088156714e+29)).*4.447070890666667e+5)./(tau_w.*2.444803076916086e+19-lt.*tau_w.*3.066951346239308e+20)).*2.0).^2.*1.447792593175879e+32-tan(atan(((lt.*3.671450002392298e+16-sqrt(lt.^2.*1.34795451200664e+33-tau_w.^2.*3.022314549036573e+27+lt.^2.*tau_w.^2.*4.75626088156714e+29)).*4.447070890666667e+5)./(tau_w.*2.444803076916086e+19-lt.*tau_w.*3.066951346239308e+20)).*2.0).^2.*5.46622816503927e+32+lt.^2.*tan(atan(((lt.*3.671450002392298e+16-sqrt(lt.^2.*1.34795451200664e+33-tau_w.^2.*3.022314549036573e+27+lt.^2.*tau_w.^2.*4.75626088156714e+29)).*4.447070890666667e+5)./(tau_w.*2.444803076916086e+19-lt.*tau_w.*3.066951346239308e+20)).*2.0).^2.*4.275634069905172e+36-tau.^2.*tan(atan(((lt.*3.671450002392298e+16-sqrt(lt.^2.*1.34795451200664e+33-tau_w.^2.*3.022314549036573e+27+lt.^2.*tau_w.^2.*4.75626088156714e+29)).*4.447070890666667e+5)./(tau_w.*2.444803076916086e+19-lt.*tau_w.*3.066951346239308e+20)).*2.0).^2.*9.586607664225985e+30-tau.^2.*9.586607664225985e+30+lt.^2.*tau.*tan(atan(((lt.*3.671450002392298e+16-sqrt(lt.^2.*1.34795451200664e+33-tau_w.^2.*3.022314549036573e+27+lt.^2.*tau_w.^2.*4.75626088156714e+29)).*4.447070890666667e+5)./(tau_w.*2.444803076916086e+19-lt.*tau_w.*3.066951346239308e+20)).*2.0).^2.*5.820228783664543e+34+lt.^2.*tau.^2.*tan(atan(((lt.*3.671450002392298e+16-sqrt(lt.^2.*1.34795451200664e+33-tau_w.^2.*3.022314549036573e+27+lt.^2.*tau_w.^2.*4.75626088156714e+29)).*4.447070890666667e+5)./(tau_w.*2.444803076916086e+19-lt.*tau_w.*3.066951346239308e+20)).*2.0).^2.*1.980704062856608e+32-5.46622816503927e+32,lt.^2.*tan(atan(((lt.*3.671450002392298e+16-sqrt(lt.^2.*1.34795451200664e+33-tau_w.^2.*3.022314549036573e+27+lt.^2.*tau_w.^2.*4.75626088156714e+29)).*4.447070890666667e+5)./(tau_w.*2.444803076916086e+19-lt.*tau_w.*3.066951346239308e+20)).*2.0).*1.710253627962069e+37+lt.^2.*tau.^2.*tan(atan(((lt.*3.671450002392298e+16-sqrt(lt.^2.*1.34795451200664e+33-tau_w.^2.*3.022314549036573e+27+lt.^2.*tau_w.^2.*4.75626088156714e+29)).*4.447070890666667e+5)./(tau_w.*2.444803076916086e+19-lt.*tau_w.*3.066951346239308e+20)).*2.0).*7.922816251426434e+32+lt.^2.*tau.*tan(atan(((lt.*3.671450002392298e+16-sqrt(lt.^2.*1.34795451200664e+33-tau_w.^2.*3.022314549036573e+27+lt.^2.*tau_w.^2.*4.75626088156714e+29)).*4.447070890666667e+5)./(tau_w.*2.444803076916086e+19-lt.*tau_w.*3.066951346239308e+20)).*2.0).*2.328091513465817e+35,tau.*2.895585186351758e+32+tau.*tan(atan(((lt.*3.671450002392298e+16-sqrt(lt.^2.*1.34795451200664e+33-tau_w.^2.*3.022314549036573e+27+lt.^2.*tau_w.^2.*4.75626088156714e+29)).*4.447070890666667e+5)./(tau_w.*2.444803076916086e+19-lt.*tau_w.*3.066951346239308e+20)).*2.0).^2.*2.895585186351758e+32+tan(atan(((lt.*3.671450002392298e+16-sqrt(lt.^2.*1.34795451200664e+33-tau_w.^2.*3.022314549036573e+27+lt.^2.*tau_w.^2.*4.75626088156714e+29)).*4.447070890666667e+5)./(tau_w.*2.444803076916086e+19-lt.*tau_w.*3.066951346239308e+20)).*2.0).^2.*1.093245633007854e+33+lt.^2.*tau.*2.328091513465817e+35-lt.^2.*tan(atan(((lt.*3.671450002392298e+16-sqrt(lt.^2.*1.34795451200664e+33-tau_w.^2.*3.022314549036573e+27+lt.^2.*tau_w.^2.*4.75626088156714e+29)).*4.447070890666667e+5)./(tau_w.*2.444803076916086e+19-lt.*tau_w.*3.066951346239308e+20)).*2.0).^2.*8.551268139810345e+36+tau.^2.*tan(atan(((lt.*3.671450002392298e+16-sqrt(lt.^2.*1.34795451200664e+33-tau_w.^2.*3.022314549036573e+27+lt.^2.*tau_w.^2.*4.75626088156714e+29)).*4.447070890666667e+5)./(tau_w.*2.444803076916086e+19-lt.*tau_w.*3.066951346239308e+20)).*2.0).^2.*1.917321532845197e+31+lt.^2.*1.710253627962069e+37+tau.^2.*1.917321532845197e+31+lt.^2.*tau.^2.*7.922816251426434e+32-lt.^2.*tau.*tan(atan(((lt.*3.671450002392298e+16-sqrt(lt.^2.*1.34795451200664e+33-tau_w.^2.*3.022314549036573e+27+lt.^2.*tau_w.^2.*4.75626088156714e+29)).*4.447070890666667e+5)./(tau_w.*2.444803076916086e+19-lt.*tau_w.*3.066951346239308e+20)).*2.0).^2.*1.164045756732909e+35-lt.^2.*tau.^2.*tan(atan(((lt.*3.671450002392298e+16-sqrt(lt.^2.*1.34795451200664e+33-tau_w.^2.*3.022314549036573e+27+lt.^2.*tau_w.^2.*4.75626088156714e+29)).*4.447070890666667e+5)./(tau_w.*2.444803076916086e+19-lt.*tau_w.*3.066951346239308e+20)).*2.0).^2.*3.961408125713217e+32+1.093245633007854e+33,lt.^2.*tan(atan(((lt.*3.671450002392298e+16-sqrt(lt.^2.*1.34795451200664e+33-tau_w.^2.*3.022314549036573e+27+lt.^2.*tau_w.^2.*4.75626088156714e+29)).*4.447070890666667e+5)./(tau_w.*2.444803076916086e+19-lt.*tau_w.*3.066951346239308e+20)).*2.0).*-1.710253627962069e+37-lt.^2.*tau.^2.*tan(atan(((lt.*3.671450002392298e+16-sqrt(lt.^2.*1.34795451200664e+33-tau_w.^2.*3.022314549036573e+27+lt.^2.*tau_w.^2.*4.75626088156714e+29)).*4.447070890666667e+5)./(tau_w.*2.444803076916086e+19-lt.*tau_w.*3.066951346239308e+20)).*2.0).*7.922816251426434e+32-lt.^2.*tau.*tan(atan(((lt.*3.671450002392298e+16-sqrt(lt.^2.*1.34795451200664e+33-tau_w.^2.*3.022314549036573e+27+lt.^2.*tau_w.^2.*4.75626088156714e+29)).*4.447070890666667e+5)./(tau_w.*2.444803076916086e+19-lt.*tau_w.*3.066951346239308e+20)).*2.0).*2.328091513465817e+35,tau.*-1.447792593175879e+32-tau.*tan(atan(((lt.*3.671450002392298e+16-sqrt(lt.^2.*1.34795451200664e+33-tau_w.^2.*3.022314549036573e+27+lt.^2.*tau_w.^2.*4.75626088156714e+29)).*4.447070890666667e+5)./(tau_w.*2.444803076916086e+19-lt.*tau_w.*3.066951346239308e+20)).*2.0).^2.*1.447792593175879e+32-tan(atan(((lt.*3.671450002392298e+16-sqrt(lt.^2.*1.34795451200664e+33-tau_w.^2.*3.022314549036573e+27+lt.^2.*tau_w.^2.*4.75626088156714e+29)).*4.447070890666667e+5)./(tau_w.*2.444803076916086e+19-lt.*tau_w.*3.066951346239308e+20)).*2.0).^2.*5.46622816503927e+32+lt.^2.*tan(atan(((lt.*3.671450002392298e+16-sqrt(lt.^2.*1.34795451200664e+33-tau_w.^2.*3.022314549036573e+27+lt.^2.*tau_w.^2.*4.75626088156714e+29)).*4.447070890666667e+5)./(tau_w.*2.444803076916086e+19-lt.*tau_w.*3.066951346239308e+20)).*2.0).^2.*4.275634069905172e+36-tau.^2.*tan(atan(((lt.*3.671450002392298e+16-sqrt(lt.^2.*1.34795451200664e+33-tau_w.^2.*3.022314549036573e+27+lt.^2.*tau_w.^2.*4.75626088156714e+29)).*4.447070890666667e+5)./(tau_w.*2.444803076916086e+19-lt.*tau_w.*3.066951346239308e+20)).*2.0).^2.*9.586607664225985e+30-tau.^2.*9.586607664225985e+30+lt.^2.*tau.*tan(atan(((lt.*3.671450002392298e+16-sqrt(lt.^2.*1.34795451200664e+33-tau_w.^2.*3.022314549036573e+27+lt.^2.*tau_w.^2.*4.75626088156714e+29)).*4.447070890666667e+5)./(tau_w.*2.444803076916086e+19-lt.*tau_w.*3.066951346239308e+20)).*2.0).^2.*5.820228783664543e+34+lt.^2.*tau.^2.*tan(atan(((lt.*3.671450002392298e+16-sqrt(lt.^2.*1.34795451200664e+33-tau_w.^2.*3.022314549036573e+27+lt.^2.*tau_w.^2.*4.75626088156714e+29)).*4.447070890666667e+5)./(tau_w.*2.444803076916086e+19-lt.*tau_w.*3.066951346239308e+20)).*2.0).^2.*1.980704062856608e+32-5.46622816503927e+32]);
    | if tau_w >= 0
    |     t2 = real(t0(4));
    | else
    |     t2 = real(t0(3));
    | end
    | inv_cog_theta1 = atan(t2).*2.0;
    | if nargout > 1
    |     t3 = lt.^2;
    |     t4 = tau.^2;
    |     t5 = tau_w.^2;
    |     t6 = tau_w.*4.0e+2;
    |     t7 = tau.*1.40737488355328e+14;
    |     t8 = tau.*2.81474976710656e+14;
    |     t9 = lt.*3.671450002392298e+16;
    |     t14 = tau.*1.447792593175879e+32;
    |     t22 = lt.*tau_w.*5.017911463213649e+3;
    |     t10 = t5.*3.022314549036573e+27;
    |     t12 = t8+2.125451466876857e+15;
    |     t13 = t7+7.590898095988775e+15;
    |     t15 = t4.*9.586607664225985e+30;
    |     t18 = t3.*1.34795451200664e+33;
    |     t19 = t3.*tau.*2.328091513465817e+35;
    |     t20 = t3.*t4.*7.922816251426434e+32;
    |     t21 = t3.*1.710253627962069e+37;
    |     t23 = -t22;
    |     t26 = t3.*t5.*4.75626088156714e+29;
    |     t11 = -t10;
    |     t16 = 1.0./t13;
    |     t17 = 1.0./t12;
    |     t24 = t6+t23;
    |     t25 = 1.0./t24;
    |     t27 = t11+t18+t26;
    |     t28 = sqrt(t27);
    |     t29 = -t28;
    |     t30 = t9+t29;
    |     t31 = (t25.*t30)./1.37438953472e+11;
    |     t32 = atan(t31);
    |     t33 = t32.*2.0;
    |     t34 = tan(t33);
    |     t35 = t34.^2;
    |     t36 = t34.^3;
    |     t37 = t35+1.0;
    |     t39 = t35.*5.46622816503927e+32;
    |     t40 = t14.*t35;
    |     t41 = t15.*t35;
    |     t42 = t3.*t35.*tau.*5.820228783664543e+34;
    |     t43 = t3.*t4.*t35.*1.980704062856608e+32;
    |     t45 = t3.*t35.*4.275634069905172e+36;
    |     t38 = 1.0./t37;
    |     t44 = -t42;
    |     t46 = -t43;
    |     t47 = -t45;
    |     et1 = t4.*1.385700562374483e+33+t34.*2.186491266015708e+34+t35.*9.713061509417766e+35+t36.*2.186491266015708e+34+tau.*1.390943230767213e+35;
    |     et2 = t3.*t34.*-3.420507255924138e+38+t4.*t34.*3.834643065690394e+32-t3.*t36.*1.710253627962069e+38+t4.*t35.*1.385700562374483e+33+t4.*t36.*3.834643065690394e+32;
    |     et3 = t34.*tau.*5.791170372703516e+33+t35.*tau.*1.390943230767213e+35+t36.*tau.*5.791170372703516e+33-t3.*t4.*t34.*1.584563250285287e+34-t3.*t4.*t36.*7.922816251426434e+33;
    |     et4 = t3.*t34.*tau.*-4.656183026931634e+36-t3.*t36.*tau.*2.328091513465817e+36+9.713061509417766e+35;
    |     et5 = t4.*2.875982299267795e+31+t19+t20+t21+t35.*1.639868449511781e+33+t42+t43+t45+tau.*4.343377779527637e+32+t4.*t35.*2.875982299267795e+31+t35.*tau.*4.343377779527637e+32;
    |     et6 = 1.639868449511781e+33;
    |     et7 = t16.*t17.*t38.*(et1+et2+et3+et4).*(-1.136363636363636e-5)-(t2.*t16.*t17.*t38.*(et5+et6))./2.2e+3+(t2.^3.*t16.*t17.*t38.*(t14+t15+t39+t40+t41+t44+t46+t47+5.46622816503927e+32))./2.2e+3;
    |     et8 = (t2.^2.*t16.*t17.*t34.*t38.*(t14+t15-t19-t20-t21+t39+t44+t46+t47+t4.*t35.*9.586607664225985e+30+t35.*tau.*1.447792593175879e+32+5.46622816503927e+32))./2.2e+3;
    |     inv_cog_delta2 = et7+et8;
    | end
    | if nargout > 2
    |     inv_cog_dtheta1 = 0.0;
    | end
    | if nargout > 3
    |     inv_cog_ddelta2 = 0.0;
    | end
    | end
